simulink model "method3"  (R2023b)
settings: Solver=VariableStepAuto  StartTime=0.0  StopTime=10.0  RelTol=1e-3
InitFcn:
  | constants_pend
values from neighbouring files (symbols this model uses):
  f = 2    [constants_pend.m]    (also in formethod3.m = u(1))
  initial = [0.5 , 5 , pi/3 , 0 ]    [constants_pend.m]
settings Model: Creator=User  LastModifiedBy=User

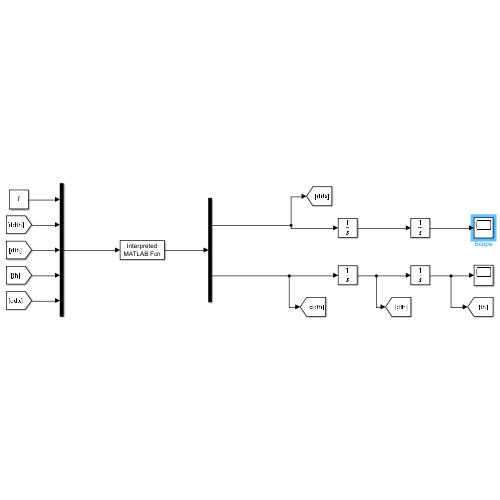
[thumbnail: Simulink's stored preview of the top-level diagram]
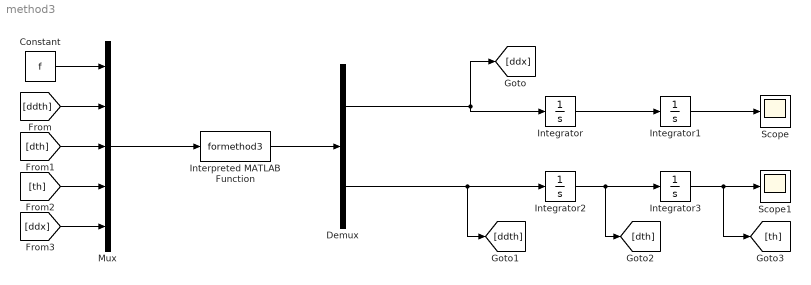
== system method3 ==
  Constant : Constant  Value=f
  Demux : Demux  Outputs=2
  Integrator : Integrator  InitialCondition=initial(2)
  Integrator1 : Integrator  InitialCondition=initial(1)
  Integrator2 : Integrator  InitialCondition=initial(4)
  Integrator3 : Integrator  InitialCondition=initial(3)
  Interpreted MATLAB Function : MATLABFcn  MATLABFcn=formethod3
  Mux : Mux  Inputs=5
  Scope : Scope
  Scope1 : Scope
  wires:
  Demux/2 -> [ddth], Integrator2/1
  Demux/1 -> Integrator/1, [ddx]
  Integrator2/1 -> [dth], Integrator3/1
  Integrator/1 -> Integrator1/1
  Integrator1/1 -> Scope/1
  Integrator3/1 -> [th], Scope1/1
  Mux/1 -> Interpreted MATLAB Function/1
  Interpreted MATLAB Function/1 -> Demux/1
  [th] -> Mux/4
  [dth] -> Mux/3
  [ddx] -> Mux/5
  [ddth] -> Mux/2
  Constant/1 -> Mux/1
